simulink model "pmsm_initial_position"  (R2022b)
settings: Solver=FixedStepAuto  StartTime=0.0  StopTime=0.6  FixedStep=0.00002  MinStep=0.00025  RelTol=1e-3
values from neighbouring files (symbols this model uses):
  B = 0.0000028    (= 2.8e-06)    [pm_params.m]
  J = 0.00016    [pm_params.m]
  Lamda_f = 0.03    [pm_params.m]
  Ld = 0.0057    [pm_params.m]
  Lq = 0.0125    [pm_params.m]
  pole = 4    [pm_params.m]
  Rs = 1.2    [pm_params.m]
settings Model: Creator=jack  LastModifiedBy=jackyeh

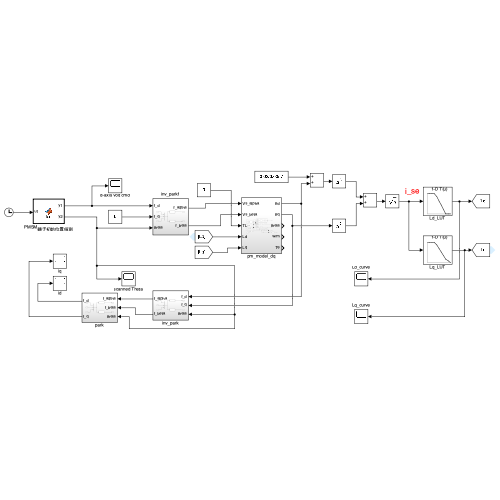
[thumbnail: Simulink's stored preview of the top-level diagram]
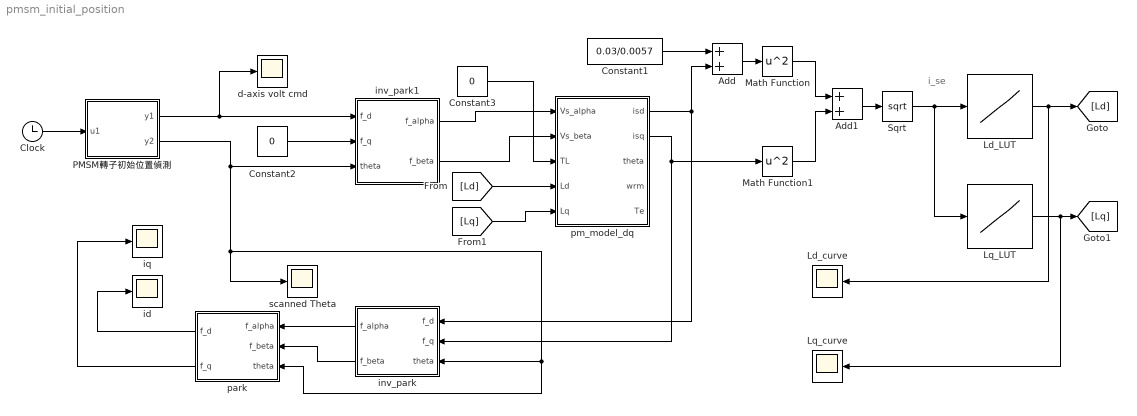
== system pmsm_initial_position ==
  note: i_se
  Add : Sum
  Add1 : Sum
  Clock : Clock
  Constant1 : Constant  Value=0.03/0.0057
  Constant2 : Constant  Value=0
  Constant3 : Constant  Value=0
  Ld_LUT : Lookup_n-D  NumberOfTableDimensions=1  BreakpointsForDimension1=[0 1 2 3 4 5 6 7 8 9 10]  Table=[0.0057 0.0057 0.0057 0.0057 0.005 0.004 0.003 0.002 0.001 0.001 0.001]  TableDataTypeStr=double  ExtrapMethod=Clip  UseLastTableValue=on  InternalRulePriority=Speed  OutDataTypeStr=double  RndMeth=Simplest
  Ld_curve : Scope
  Lq_LUT : Lookup_n-D  NumberOfTableDimensions=1  BreakpointsForDimension1=[0 1 2 3 4 5 6 7 8 9 10]  Table=[0.0125 0.0125 0.0125 0.0125 0.011 0.009 0.007 0.005 0.003 0.002 0.001]  TableDataTypeStr=double  ExtrapMethod=Clip  UseLastTableValue=on  InternalRulePriority=Speed  OutDataTypeStr=double  RndMeth=Simplest
  Lq_curve : Scope
  Math Function : Math  Operator=square
  Math Function1 : Math  Operator=square
  PMSM轉子初始位置偵測 : MATLAB Function  TreatAsAtomicUnit=on
  Sqrt : Sqrt
  d-axis volt cmd : Scope
  id : Scope
  inv_park : Subsystem
  inv_park1 : Subsystem
  iq : Scope
  park : Subsystem
  pm_model_dq : Subsystem
  scanned Theta : Scope
  wires:
  pm_model_dq/2(isq) -> Math Function1/1, inv_park/2(f_q)
  pm_model_dq/1(isd) -> inv_park/1(f_d), Add/2
  Constant3/1 -> pm_model_dq/3(TL)
  PMSM轉子初始位置偵測/2(y2) -> inv_park/3(theta), park/3(theta), scanned Theta/1, inv_park1/3(theta)
  inv_park/1(f_alpha) -> park/1(f_alpha)
  inv_park/2(f_beta) -> park/2(f_beta)
  park/1(f_d) -> id/1
  park/2(f_q) -> iq/1
  inv_park1/1(f_alpha) -> pm_model_dq/1(Vs_alpha)
  inv_park1/2(f_beta) -> pm_model_dq/2(Vs_beta)
  Clock/1 -> PMSM轉子初始位置偵測/1(u1)
  PMSM轉子初始位置偵測/1(y1) -> d-axis volt cmd/1, inv_park1/1(f_d)
  Constant2/1 -> inv_park1/2(f_q)
  Constant1/1 -> Add/1
  Add/1 -> Math Function/1
  Math Function/1 -> Add1/1
  Math Function1/1 -> Add1/2
  Add1/1 -> Sqrt/1
  Sqrt/1 -> Lq_LUT/1, Ld_LUT/1
  Ld_LUT/1 -> [Ld], Ld_curve/1
  Lq_LUT/1 -> Lq_curve/1, [Lq]
  [Ld] -> pm_model_dq/4(Ld)
  [Lq] -> pm_model_dq/5(Lq)

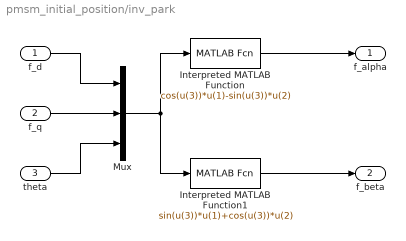
== system pmsm_initial_position/inv_park ==
  f_d : Inport
  f_q : Inport  Port=2
  theta : Inport  Port=3
  Interpreted MATLAB Function : MATLABFcn  MATLABFcn=cos(u(3))*u(1)-sin(u(3))*u(2)
  Interpreted MATLAB Function1 : MATLABFcn  MATLABFcn=sin(u(3))*u(1)+cos(u(3))*u(2)
  Mux : Mux  Inputs=3
  f_alpha : Outport
  f_beta : Outport  Port=2
  wires:
  Interpreted MATLAB Function/1 -> f_alpha/1
  f_d/1 -> Mux/1
  Mux/1 -> Interpreted MATLAB Function1/1, Interpreted MATLAB Function/1
  Interpreted MATLAB Function1/1 -> f_beta/1
  theta/1 -> Mux/3
  f_q/1 -> Mux/2

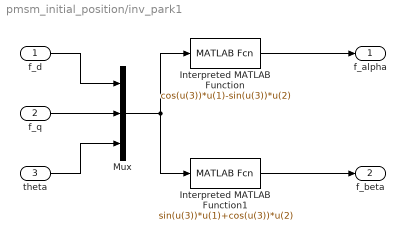
== system pmsm_initial_position/inv_park1 ==
  f_d : Inport
  f_q : Inport  Port=2
  theta : Inport  Port=3
  Interpreted MATLAB Function : MATLABFcn  MATLABFcn=cos(u(3))*u(1)-sin(u(3))*u(2)
  Interpreted MATLAB Function1 : MATLABFcn  MATLABFcn=sin(u(3))*u(1)+cos(u(3))*u(2)
  Mux : Mux  Inputs=3
  f_alpha : Outport
  f_beta : Outport  Port=2
  wires:
  f_q/1 -> Mux/2
  theta/1 -> Mux/3
  Interpreted MATLAB Function1/1 -> f_beta/1
  Mux/1 -> Interpreted MATLAB Function/1, Interpreted MATLAB Function1/1
  f_d/1 -> Mux/1
  Interpreted MATLAB Function/1 -> f_alpha/1

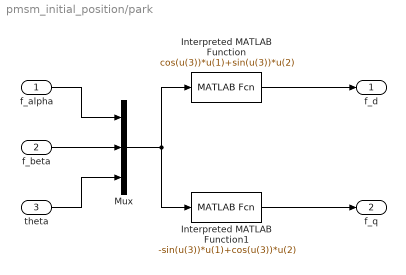
== system pmsm_initial_position/park ==
  f_alpha : Inport
  f_beta : Inport  Port=2
  theta : Inport  Port=3
  Interpreted MATLAB Function : MATLABFcn  MATLABFcn=cos(u(3))*u(1)+sin(u(3))*u(2)
  Interpreted MATLAB Function1 : MATLABFcn  MATLABFcn=-sin(u(3))*u(1)+cos(u(3))*u(2)
  Mux : Mux  Inputs=3
  f_d : Outport
  f_q : Outport  Port=2
  wires:
  Interpreted MATLAB Function/1 -> f_d/1
  f_alpha/1 -> Mux/1
  Mux/1 -> Interpreted MATLAB Function1/1, Interpreted MATLAB Function/1
  Interpreted MATLAB Function1/1 -> f_q/1
  theta/1 -> Mux/3
  f_beta/1 -> Mux/2

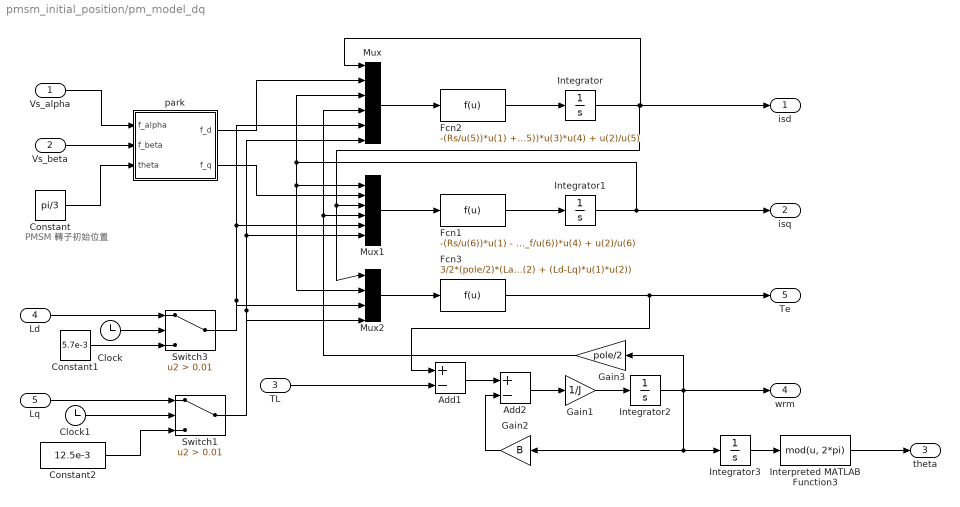
== system pmsm_initial_position/pm_model_dq ==
  note: PMSM 轉子初始位置
  Vs_alpha : Inport
  Vs_beta : Inport  Port=2
  TL : Inport  Port=3
  Ld : Inport  Port=4
  Lq : Inport  Port=5
  Add1 : Sum  Inputs=+-
  Add2 : Sum  Inputs=+-
  Clock : Clock
  Clock1 : Clock
  Constant : Constant  Value=pi/3
  Constant1 : Constant  Value=5.7e-3
  Constant2 : Constant  Value=12.5e-3
  Fcn1 : Fcn  Expr=-(Rs/u(6))*u(1) - (u(5)/u(6))*u(3)*u(4) - (Lamda_f/u(6))*u(4) + u(2)/u(6)
  Fcn2 : Fcn  Expr=-(Rs/u(5))*u(1) + (u(6)/u(5))*u(3)*u(4) + u(2)/u(5)
  Fcn3 : Fcn  Expr=3/2*(pole/2)*(Lamda_f*u(2) + (Ld-Lq)*u(1)*u(2))
  Gain1 : Gain  Gain=1/J
  Gain2 : Gain  Gain=B
  Gain3 : Gain  Gain=pole/2
  Integrator{,1..3} (4 alike) : Integrator
  Interpreted MATLAB Function3 : MATLABFcn  MATLABFcn=mod(u, 2*pi)
  Mux : Mux  Inputs=6
  Mux1 : Mux  Inputs=6
  Mux2 : Mux
  Switch1 : Switch  Criteria=u2 > Threshold  Threshold=0.01  SaturateOnIntegerOverflow=off  InputSameDT=off
  Switch3 : Switch  Criteria=u2 > Threshold  Threshold=0.01  SaturateOnIntegerOverflow=off  InputSameDT=off
  park : Subsystem
  isd : Outport
  isq : Outport  Port=2
  theta : Outport  Port=3
  wrm : Outport  Port=4
  Te : Outport  Port=5
  wires:
  Mux/1 -> Fcn2/1
  Fcn1/1 -> Integrator1/1
  TL/1 -> Add1/2
  Integrator1/1 -> isq/1, Mux/3, Mux2/2, Mux1/1
  Fcn3/1 -> Te/1, Add1/1
  Gain3/1 -> Mux/4, Mux1/4
  Add2/1 -> Gain1/1
  Gain1/1 -> Integrator2/1
  Add1/1 -> Add2/1
  Mux2/1 -> Fcn3/1
  Fcn2/1 -> Integrator/1
  Integrator/1 -> isd/1, Mux/1, Mux2/1, Mux1/3
  Integrator2/1 -> wrm/1, Gain3/1, Integrator3/1, Gain2/1
  Interpreted MATLAB Function3/1 -> theta/1
  Mux1/1 -> Fcn1/1
  Gain2/1 -> Add2/2
  Integrator3/1 -> Interpreted MATLAB Function3/1
  park/1(f_d) -> Mux/2
  park/2(f_q) -> Mux1/2
  Vs_alpha/1 -> park/1(f_alpha)
  Vs_beta/1 -> park/2(f_beta)
  Constant/1 -> park/3(theta)
  Clock/1 -> Switch3/2
  Constant1/1 -> Switch3/3
  Constant2/1 -> Switch1/3
  Ld/1 -> Switch3/1
  Switch3/1 -> Mux1/5, Mux/5, Mux2/3
  Switch1/1 -> Mux2/4, Mux1/6, Mux/6
  Clock1/1 -> Switch1/2
  Lq/1 -> Switch1/1

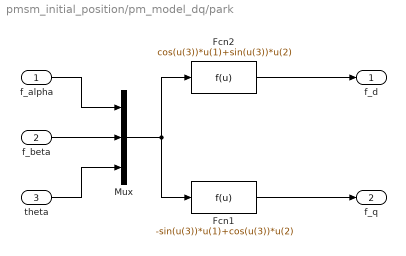
== system pmsm_initial_position/pm_model_dq/park ==
  f_alpha : Inport
  f_beta : Inport  Port=2
  theta : Inport  Port=3
  Fcn1 : Fcn  Expr=-sin(u(3))*u(1)+cos(u(3))*u(2)
  Fcn2 : Fcn  Expr=cos(u(3))*u(1)+sin(u(3))*u(2)
  Mux : Mux  Inputs=3
  f_d : Outport
  f_q : Outport  Port=2
  wires:
  Fcn2/1 -> f_d/1
  f_alpha/1 -> Mux/1
  Mux/1 -> Fcn1/1, Fcn2/1
  Fcn1/1 -> f_q/1
  theta/1 -> Mux/3
  f_beta/1 -> Mux/2

== matlab function pmsm_initial_position/PMSM轉子初始位置偵測 ==
  data: u1 input; y1 output; y2 output
function [y1, y2] = fcn(u1)
    Ts = 1e-4;
    theta_V=0:pi/12:2*pi;
    Um = 10;
    n=5; m=300;
    period = (n+m)*Ts;
    a = floor(u1/period); 
    b = mod(u1, period);
    if((u1 <= (a*period + n*Ts)) && (a<25))
      y1 = Um;
      y2 = theta_V(a+1);
    else
      y1 = 0;
      y2 = theta_V(a+1);
    end
